simulink model "FilterSimulation"  (Simulink 8.5)
settings: Solver=ode45  StartTime=0.0  StopTime=10.0  RelTol=1e-3
values from neighbouring files (symbols this model uses):
  Ks = 0.5149 * v - 0.1925    (= 0.52836)    [steeringStepResponse.m]
settings Model: Creator=rdestr15  LastModifiedBy=Amalie
settings DebuggingCC: SolverPrmCheckMsg=warning  FcnCallInpInsideContextMsg=EnableAllAsWarning
settings GRTTargetCC: CombineOutputUpdateFcns=on  GRTInterface=off

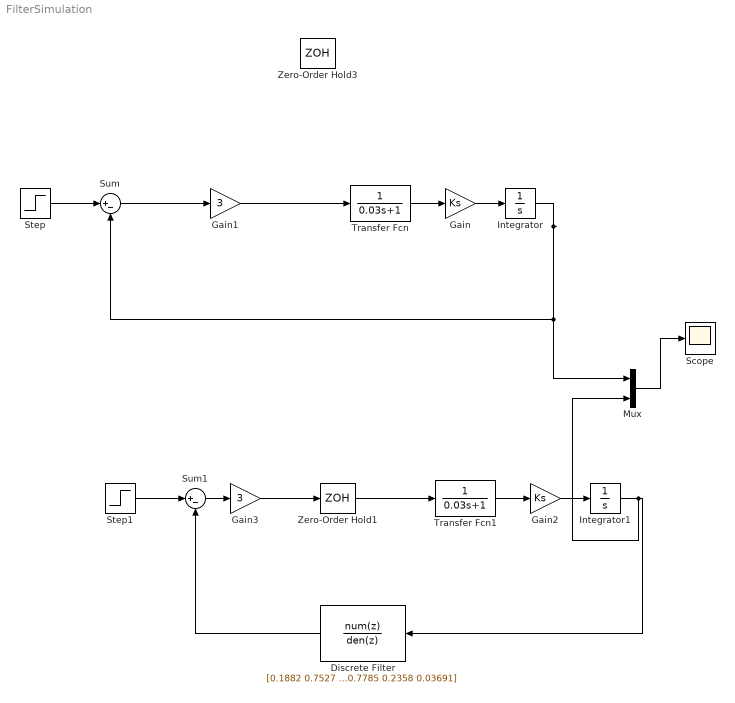
== system FilterSimulation ==
  Discrete Filter : DiscreteFilter  Numerator=[0.1882 0.7527 1.129 0.7527 0.1882]  Denominator=[1 0.9595 0.7785 0.2358 0.03691]  InputProcessing=Columns as channels (frame based)  FilterStructure=Direct form II transposed  SampleTime=0.015  a0EqualsOne=on
  Gain : Gain  Gain=Ks
  Gain1 : Gain  Gain=3
  Gain2 : Gain  Gain=Ks
  Gain3 : Gain  Gain=3
  Integrator : Integrator
  Integrator1 : Integrator
  Mux : Mux  Inputs=2
  Scope : Scope
  Step : Step  Time=5  Before=1360  After=1670  SampleTime=0
  Step1 : Step  Time=5  Before=1360  After=1670  SampleTime=0
  Sum : Sum  Inputs=|+-
  Sum1 : Sum  Inputs=|+-
  Transfer Fcn : TransferFcn  Denominator=[0.03 1]
  Transfer Fcn1 : TransferFcn  Denominator=[0.03 1]
  Zero-Order Hold1 : ZeroOrderHold  SampleTime=0.015
  Zero-Order Hold3 : ZeroOrderHold  SampleTime=0.015
  wires:
  Step/1 -> Sum/1
  Gain/1 -> Integrator/1
  Integrator/1 -> Mux/1, Sum/2
  Sum/1 -> Gain1/1
  Transfer Fcn/1 -> Gain/1
  Step1/1 -> Sum1/1
  Gain2/1 -> Integrator1/1
  Integrator1/1 -> Mux/2, Discrete Filter/1
  Sum1/1 -> Gain3/1
  Transfer Fcn1/1 -> Gain2/1
  Gain3/1 -> Zero-Order Hold1/1
  Zero-Order Hold1/1 -> Transfer Fcn1/1
  Discrete Filter/1 -> Sum1/2
  Mux/1 -> Scope/1
  Gain1/1 -> Transfer Fcn/1
